simulink model "cmd"  (R2018b)
settings: Solver=VariableStepAuto  StartTime=0.0  StopTime=10  RelTol=1e-3
settings Model: Creator=USER  LastModifiedBy=USER

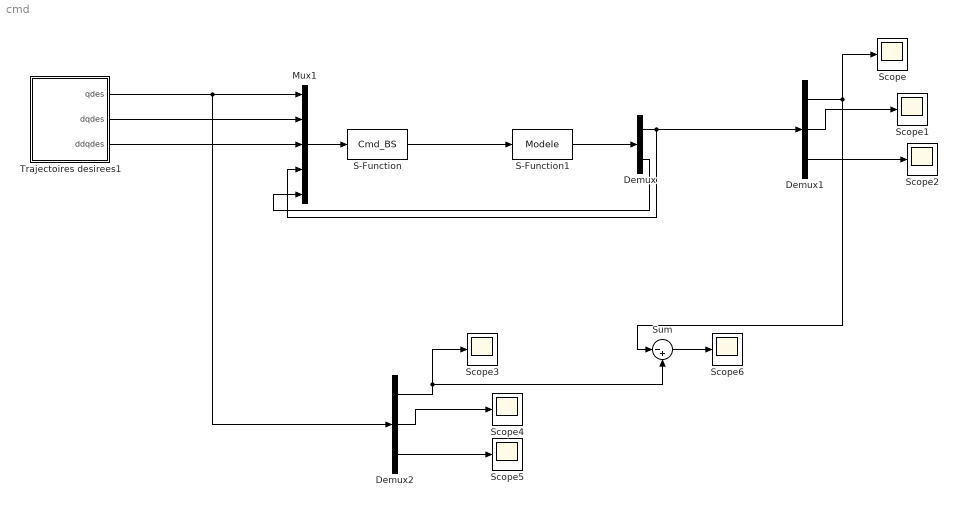
== system cmd ==
  Demux : Demux  Outputs=2
  Demux1 : Demux  Outputs=3
  Demux2 : Demux  Outputs=3
  Mux1 : Mux  Inputs=5
  S-Function : S-Function  FunctionName=Cmd_BS  SFunctionDeploymentMode=off  EnableBusSupport=off
  S-Function1 : S-Function  FunctionName=Modele  SFunctionDeploymentMode=off  EnableBusSupport=off
  Scope{,1..6} (7 alike) : Scope
  Sum : Sum  Inputs=|-+
  Trajectoires desirees1 : Subsystem
  wires:
  Mux1/1 -> S-Function/1
  S-Function/1 -> S-Function1/1
  S-Function1/1 -> Demux/1
  Demux/2 -> Mux1/5
  Trajectoires desirees1/2(dqdes) -> Mux1/2
  Trajectoires desirees1/3(ddqdes) -> Mux1/3
  Demux1/3 -> Scope2/1
  Demux1/1 -> Scope/1, Sum/1
  Demux/1 -> Demux1/1, Mux1/4
  Demux2/1 -> Sum/2, Scope3/1
  Demux2/3 -> Scope5/1
  Trajectoires desirees1/1(qdes) -> Mux1/1, Demux2/1
  Demux2/2 -> Scope4/1
  Demux1/2 -> Scope1/1
  Sum/1 -> Scope6/1

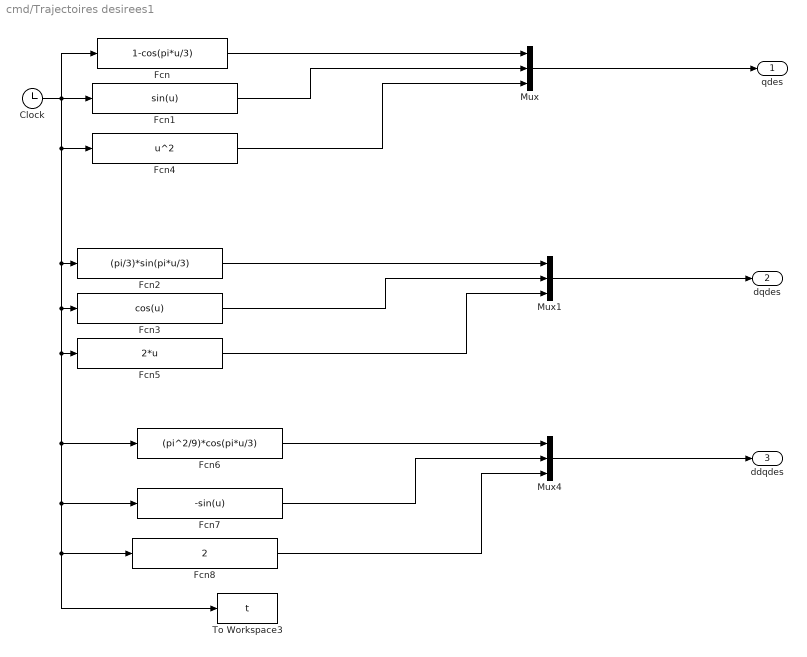
== system cmd/Trajectoires desirees1 ==
  Clock : Clock
  Fcn : Fcn  Expr=1-cos(pi*u/3)
  Fcn1 : Fcn  Expr=sin(u)
  Fcn2 : Fcn  Expr=(pi/3)*sin(pi*u/3)
  Fcn3 : Fcn  Expr=cos(u)
  Fcn4 : Fcn  Expr=u^2
  Fcn5 : Fcn  Expr=2*u
  Fcn6 : Fcn  Expr=(pi^2/9)*cos(pi*u/3)
  Fcn7 : Fcn  Expr=-sin(u)
  Fcn8 : Fcn  Expr=2
  Mux : Mux  Inputs=3
  Mux1 : Mux  Inputs=3
  Mux4 : Mux  Inputs=3
  To Workspace3 : ToWorkspace  VariableName=t  SampleTime=-1
  qdes : Outport
  dqdes : Outport  Port=2
  ddqdes : Outport  Port=3
  wires:
  Mux1/1 -> dqdes/1
  Mux/1 -> qdes/1
  Mux4/1 -> ddqdes/1
  Fcn/1 -> Mux/1
  Fcn4/1 -> Mux/3
  Fcn1/1 -> Mux/2
  Fcn2/1 -> Mux1/1
  Fcn3/1 -> Mux1/2
  Fcn5/1 -> Mux1/3
  Clock/1 -> Fcn5/1, Fcn6/1, Fcn7/1, To Workspace3/1, Fcn8/1, Fcn3/1, Fcn2/1, Fcn4/1, Fcn/1, Fcn1/1
  Fcn6/1 -> Mux4/1
  Fcn7/1 -> Mux4/2
  Fcn8/1 -> Mux4/3
